simulink model "EMPC_Simple"  (R2020a)
settings: Solver=FixedStepDiscrete  StartTime=0.0  StopTime=800  FixedStep=Ts  RelTol=1e-3
values from neighbouring files (symbols this model uses):
  filter_d = c2d(filter,Ts)    [Init.m]
  Kopt = 1/2*Parameters.rho*pi*Parameters.R^5*maxCp/Parameters.G^3/TSR_opt^3/Parameters.Effic    [Init.m]
  Parameters =     [Parameters.mat]
  Pitch_opt = Yq(JJ(III),III)    [Init.m]    (also in Plot_Cp_Cq.m)
  Ts = 0.5; Parameters.Ts=Ts    [Init.m]
undefined symbols (not defined in the file or in its folder): EMPCController_Basic
libraries: simulink x1
settings Model: Creator=jwvanwingerden  LastModifiedBy=jwvanwingerden

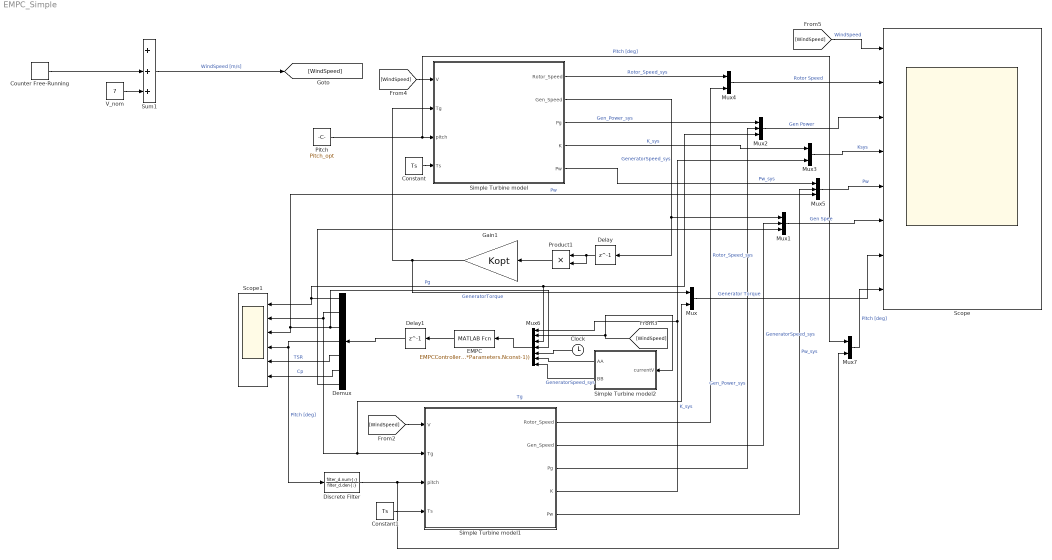
== system EMPC_Simple ==
  Clock : Clock
  Constant : Constant  Value=Ts  SampleTime=Ts
  Constant1 : Constant  Value=Ts  SampleTime=Ts
  Counter Free-Running : simulink/Sources/Counter Free-Running  NumBits=16  tsamp=50
  Delay : Delay  DelayLength=1  InitialCondition=0
  Delay1 : Delay  DelayLength=1  InitialCondition=0
  Demux : Demux  Outputs=7
  Discrete Filter : DiscreteFilter  Numerator=filter_d.num{:}  Denominator=filter_d.den{:}
  EMPC : MATLABFcn  MATLABFcn=EMPCController_Basic(u(1),u(2),u(3),u(4),u(5),u(6:1:6+Parameters.Nconst-1),u(6+Parameters.Nconst:1:6+2*Parameters.Nconst-1))  SampleTime=Ts
  Gain1 : Gain  Gain=Kopt
  Mux{,3..4,7} (4 alike) : Mux  Inputs=2
  Mux1 : Mux  Inputs=3
  Mux2 : Mux  Inputs=3
  Mux5 : Mux  Inputs=3
  Mux6 : Mux  Inputs=7
  Pitch : Constant  Value=Pitch_opt
  Product1 : Product
  Scope : Scope  NumInputPorts=8
  Scope1 : Scope  NumInputPorts=6
  Simple Turbine model : MATLAB Function  TreatAsAtomicUnit=on  SystemSampleTime=Ts
  Simple Turbine model1 : MATLAB Function  TreatAsAtomicUnit=on  SystemSampleTime=Ts
  Simple Turbine model2 : MATLAB Function  TreatAsAtomicUnit=on  SystemSampleTime=Ts
  Sum1 : Sum  Inputs=+++
  V_nom : Constant  Value=7
  wires:
  V_nom/1 -> Sum1/3
  Product1/1 -> Gain1/1
  Gain1/1 -> Mux/1, Simple Turbine model/2(Tg)  "GeneratorTorque"
  Constant/1 -> Simple Turbine model/4(Ts)
  Pitch/1 -> Mux7/1, Simple Turbine model/3(pitch)  "Pitch [deg]"
  Delay/1 -> Product1/2, Product1/1
  Mux2/1 -> Scope/3  "Gen Power"
  Simple Turbine model/2(Gen_Speed) -> Mux1/1, Delay/1  "GeneratorSpeed_sys"
  Mux1/1 -> Scope/6  "Gen Spee"
  Mux/1 -> Scope/7  "Generator Torque"
  Simple Turbine model/3(Pg) -> Mux2/1  "Gen_Power_sys"
  Simple Turbine model/4(K) -> Mux3/1  "K_sys"
  Mux3/1 -> Scope/4  "Ksys"
  Mux4/1 -> Scope/2  "Rotor Speed"
  Simple Turbine model/1(Rotor_Speed) -> Mux4/1  "Rotor_Speed_sys"
  Mux5/1 -> Scope/5  "Pw"
  Simple Turbine model/5(Pw) -> Mux5/1  "Pw_sys"
  Mux6/1 -> EMPC/1
  EMPC/1 -> Delay1/1
  Demux/2 -> Mux/2, Simple Turbine model1/2(Tg), Scope1/2  "Tg"
  Demux/1 -> Scope1/1, Mux2/3, Mux6/3  "Pg"
  Demux/3 -> Mux6/4, Scope1/3, Mux5/3  "Pw"
  [WindSpeed] -> Simple Turbine model/1(V)
  [WindSpeed] -> Scope/1  "WindSpeed"
  [WindSpeed] -> Simple Turbine model1/1(V)
  Simple Turbine model1/4(K) -> Mux6/1, Mux3/2  "K_sys"
  [WindSpeed] -> Simple Turbine model2/1(currentV), Mux6/2
  Simple Turbine model1/1(Rotor_Speed) -> Mux4/2  "Rotor_Speed_sys"
  Simple Turbine model1/3(Pg) -> Mux2/2  "Gen_Power_sys"
  Simple Turbine model1/5(Pw) -> Mux5/2  "Pw_sys"
  Constant1/1 -> Simple Turbine model1/4(Ts)
  Delay1/1 -> Demux/1
  Simple Turbine model1/2(Gen_Speed) -> Mux1/2  "GeneratorSpeed_sys"
  Demux/4 -> Discrete Filter/1, Scope1/4  "Pitch [deg]"
  Demux/5 -> Scope1/5  "TSR"
  Demux/6 -> Scope1/6  "Cp"
  Mux7/1 -> Scope/8  "Pitch [deg]"
  Sum1/1 -> [WindSpeed]  "WindSpeed [m/s]"
  Demux/7 -> Mux1/3
  Simple Turbine model2/1(AA) -> Mux6/6
  Simple Turbine model2/2(BB) -> Mux6/7  "GeneratorSpeed_sys"
  Discrete Filter/1 -> Mux7/2, Simple Turbine model1/3(pitch)
  Counter Free-Running/1 -> Sum1/2
  Clock/1 -> Mux6/5

== matlab function EMPC_Simple/Simple Turbine model1 ==
  data: V input; Rotor_Speed output; Tg input; pitch input; Ts input; Gen_Speed output; Pg output; Parameters parameter; K output; Pw output
function [Rotor_Speed,Gen_Speed,Pg,K,Pw]  = fcn(V,Tg,pitch,Ts, Parameters)

persistent omega2 
if isempty(omega2);
    omega2=0.1*2*pi;
end

omega_p=omega2;

TSR=omega_p*Parameters.R/V;

Cq = interp2(Parameters.Rotor_Lamda,Parameters.Rotor_Pitch,Parameters.Rotor_cQ,TSR,pitch,'cubic');
Ta = 1/2*Parameters.rho*pi*Parameters.R^3*Cq*V^2;
omega2=omega_p+Ts*(1/Parameters.J*(Ta-Parameters.Effic*Tg*Parameters.G))

%% output
Rotor_Speed=omega2;
Gen_Speed=omega2*Parameters.G;
Pg=omega2*Parameters.G*Tg*Parameters.Effic;
K=1/2*Gen_Speed.^2*Parameters.J;
Pw=Ta/Parameters.G*Gen_Speed;

== matlab function EMPC_Simple/Simple Turbine model2 ==
  settings: updateMethod=DISCRETE  sampleTime=Ts
  data: currentV input size=1; AA output size=[Parameters.Nconst,1]; BB output size=[Parameters.Nconst,1]; Parameters parameter
function [AA,BB]  = fcn(currentV, Parameters)

AA=zeros(Parameters.Nconst,1);
BB=zeros(Parameters.Nconst,1);

%qq=find(sign(diff(sign(Parameters.BOUNDPW.V-currentV))),1);
[~,qq]=max(((Parameters.BOUNDPW.V-currentV)>=0)*-20+Parameters.BOUNDPW.V-currentV);
fraction=1-(currentV-Parameters.BOUNDPW.V(qq))/(Parameters.BOUNDPW.V(qq+1)-Parameters.BOUNDPW.V(qq));



AA=(Parameters.BOUNDPW.Ac(:,qq)*fraction+Parameters.BOUNDPW.Ac(:,qq+1)*(1-fraction));
BB=(Parameters.BOUNDPW.Bc(:,qq)*fraction+Parameters.BOUNDPW.Bc(:,qq+1)*(1-fraction));

== matlab function EMPC_Simple/Simple Turbine model ==
  data: V input; Rotor_Speed output; Tg input; pitch input; Ts input; Gen_Speed output; Pg output; Parameters parameter; K output; Pw output
function [Rotor_Speed,Gen_Speed,Pg,K,Pw]  = fcn(V,Tg,pitch,Ts, Parameters)

persistent omega 
if isempty(omega);
    omega=0.1*2*pi;
end

omega_p=omega;

TSR=omega_p*Parameters.R/V;

Cq = interp2(Parameters.Rotor_Lamda,Parameters.Rotor_Pitch,Parameters.Rotor_cQ,TSR,pitch,'cubic');
Ta = 1/2*Parameters.rho*pi*Parameters.R^3*Cq*V^2;
omega=omega_p+Ts*(1/Parameters.J*(Ta-Parameters.Effic*Tg*Parameters.G))

%% output
Rotor_Speed=omega;
Gen_Speed=omega*Parameters.G;
Pg=omega*Parameters.G*Tg*Parameters.Effic;
K=1/2*Gen_Speed.^2*Parameters.J;
Pw=Ta/Parameters.G*Gen_Speed;
